simulink library "MASS"  (R2016b)
settings: Solver=VariableStepAuto  StartTime=0.0  StopTime=10.0  RelTol=1e-3
libraries: aerolibutil x2, aerolibtransform2 x2
settings Model: Creator=Andrew  LastModifiedBy=Andrew

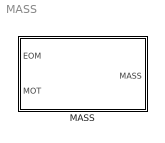
== system MASS ==
  MASS : Subsystem

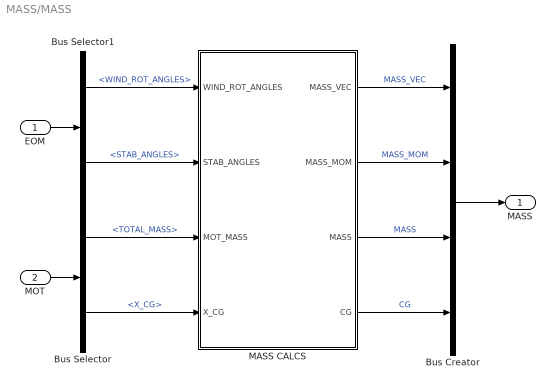
== system MASS/MASS ==
  EOM : Inport
  MOT : Inport  Port=2
  Bus Creator : BusCreator  Inputs=4
  Bus Selector : BusSelector  OutputSignals=TOTAL_MASS,X_CG
  Bus Selector1 : BusSelector  OutputSignals=WIND_ROT_ANGLES,STAB_ANGLES
  MASS CALCS : Subsystem
  MASS : Outport
  wires:
  Bus Selector1/2 -> MASS CALCS/2(STAB_ANGLES)  "<STAB_ANGLES>"
  MOT/1 -> Bus Selector/1
  Bus Selector/1 -> MASS CALCS/3(MOT_MASS)  "<TOTAL_MASS>"
  Bus Selector/2 -> MASS CALCS/4(X_CG)  "<X_CG>"
  EOM/1 -> Bus Selector1/1
  MASS CALCS/3(MASS) -> Bus Creator/3  "MASS"
  MASS CALCS/2(MASS_MOM) -> Bus Creator/2  "MASS_MOM"
  MASS CALCS/1(MASS_VEC) -> Bus Creator/1  "MASS_VEC"
  MASS CALCS/4(CG) -> Bus Creator/4  "CG"
  Bus Creator/1 -> MASS/1
  Bus Selector1/1 -> MASS CALCS/1(WIND_ROT_ANGLES)  "<WIND_ROT_ANGLES>"

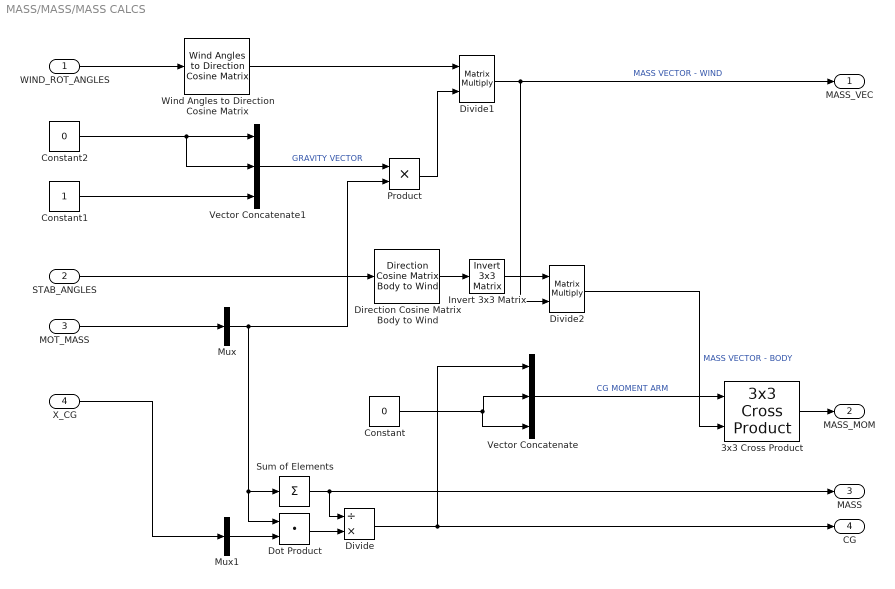
== system MASS/MASS/MASS CALCS ==
  WIND_ROT_ANGLES : Inport
  STAB_ANGLES : Inport  Port=2
  MOT_MASS : Inport  Port=3
  X_CG : Inport  Port=4
  3x3 Cross Product : aerolibutil/3x3 Cross Product
  Constant : Constant  Value=0
  Constant1 : Constant
  Constant2 : Constant  Value=0
  Direction Cosine Matrix Body to Wind : aerolibtransform2/Direction Cosine Matrix Body to Wind
  Divide : Product  Inputs=/*
  Divide1 : Product  Inputs=**  Multiplication=Matrix(*)
  Divide2 : Product  Inputs=**  Multiplication=Matrix(*)
  Dot Product : DotProduct  InputSameDT=on  OutDataTypeStr=Inherit: Inherit via internal rule
  Invert 3x3 Matrix : aerolibutil/Invert  3x3 Matrix
  Mux : Mux  Inputs=1
  Mux1 : Mux  Inputs=1
  Product : Product
  Sum of Elements : Sum  Inputs=+
  Vector Concatenate : Concatenate  NumInputs=3
  Vector Concatenate1 : Concatenate  NumInputs=3
  Wind Angles to Direction Cosine Matrix : aerolibtransform2/Wind Angles to  Direction Cosine Matrix
  MASS_VEC : Outport
  MASS_MOM : Outport  Port=2
  MASS : Outport  Port=3
  CG : Outport  Port=4
  wires:
  MOT_MASS/1 -> Mux/1
  X_CG/1 -> Mux1/1
  Mux1/1 -> Dot Product/2
  Mux/1 -> Sum of Elements/1, Dot Product/1, Product/2
  Dot Product/1 -> Divide/2
  Divide/1 -> Vector Concatenate/1, CG/1
  Sum of Elements/1 -> MASS/1, Divide/1
  Constant/1 -> Vector Concatenate/3, Vector Concatenate/2
  3x3 Cross Product/1 -> MASS_MOM/1
  Vector Concatenate/1 -> 3x3 Cross Product/1  "CG MOMENT ARM"
  Constant2/1 -> Vector Concatenate1/2, Vector Concatenate1/1
  Vector Concatenate1/1 -> Product/1  "GRAVITY VECTOR"
  WIND_ROT_ANGLES/1 -> Wind Angles to Direction Cosine Matrix/1
  Wind Angles to Direction Cosine Matrix/1 -> Divide1/1
  Product/1 -> Divide1/2
  Direction Cosine Matrix Body to Wind/1 -> Invert 3x3 Matrix/1
  Invert 3x3 Matrix/1 -> Divide2/1
  Divide1/1 -> MASS_VEC/1, Divide2/2  "MASS VECTOR - WIND"
  Divide2/1 -> 3x3 Cross Product/2  "MASS VECTOR - BODY"
  STAB_ANGLES/1 -> Direction Cosine Matrix Body to Wind/1
  Constant1/1 -> Vector Concatenate1/3
